simulink model "Microgrid_W"  (R2020a)
settings: Solver=ode15s  StartTime=0  StopTime=1440*1  MaxStep=1  RelTol=1e-3
libraries: simulink x4214, powerlib x685, simulink_extras x28, Microgrid_Library x18, powerlib_meascontrol x12
(part 37 of 48)

== system Microgrid_W/House 5 W1/Kettle/D4 ==
  Add : Sum  Inputs=+++
  Clock : Clock
  Compare To Zero : simulink/Logic and Bit Operations/Compare To Zero  relop=>  OutDataTypeStr=boolean
  Compare To Zero1 : simulink/Logic and Bit Operations/Compare To Zero  relop=>  OutDataTypeStr=boolean
  Compare To Zero2 : simulink/Logic and Bit Operations/Compare To Zero  relop=>  OutDataTypeStr=boolean
  Constant : Constant
  Constant{1..2,5,8} (4 alike) : Constant  Value=0
  Constant3 : Constant  Value=Jug_On_1
  Constant4 : Constant
  Constant6 : Constant  Value=Jug_On_2
  Constant7 : Constant
  Constant9 : Constant  Value=Jug_On_3
  Gain : Gain  Gain=t
  Interval Test : simulink/Logic and Bit Operations/Interval Test  IntervalClosedRight=on  uplimit=Jug_On_1+180+86400*3  IntervalClosedLeft=on  lowlimit=Jug_On_1+86400*3  OutDataTypeStr=boolean
  Interval Test1 : simulink/Logic and Bit Operations/Interval Test  IntervalClosedRight=on  uplimit=Jug_On_2+180+86400*3  IntervalClosedLeft=on  lowlimit=Jug_On_2+86400*3  OutDataTypeStr=boolean
  Interval Test2 : simulink/Logic and Bit Operations/Interval Test  IntervalClosedRight=on  uplimit=Jug_On_3+180+86400*3  IntervalClosedLeft=on  lowlimit=Jug_On_3+86400*3  OutDataTypeStr=boolean
  Switch{,1..5} (6 alike) : Switch  Criteria=u2 > Threshold  Threshold=0.5
  Out1 : Outport  VectorParamsAs1DForOutWhenUnconnected=off
  wires:
  Clock/1 -> Gain/1
  Interval Test/1 -> Switch/2
  Constant1/1 -> Switch3/3, Switch2/3, Switch/3
  Gain/1 -> Interval Test2/1, Interval Test1/1, Interval Test/1
  Constant3/1 -> Compare To Zero/1
  Constant/1 -> Switch1/1
  Constant2/1 -> Switch1/3
  Compare To Zero/1 -> Switch1/2
  Switch1/1 -> Switch/1
  Interval Test1/1 -> Switch2/2
  Interval Test2/1 -> Switch3/2
  Constant6/1 -> Compare To Zero1/1
  Constant4/1 -> Switch4/1
  Constant5/1 -> Switch4/3
  Compare To Zero1/1 -> Switch4/2
  Constant9/1 -> Compare To Zero2/1
  Constant7/1 -> Switch5/1
  Constant8/1 -> Switch5/3
  Compare To Zero2/1 -> Switch5/2
  Switch4/1 -> Switch2/1
  Switch5/1 -> Switch3/1
  Switch/1 -> Add/1
  Switch2/1 -> Add/2
  Switch3/1 -> Add/3
  Add/1 -> Out1/1

== system Microgrid_W/House 5 W1/Kettle/D5 ==
  Add : Sum  Inputs=+++
  Clock : Clock
  Compare To Zero : simulink/Logic and Bit Operations/Compare To Zero  relop=>  OutDataTypeStr=boolean
  Compare To Zero1 : simulink/Logic and Bit Operations/Compare To Zero  relop=>  OutDataTypeStr=boolean
  Compare To Zero2 : simulink/Logic and Bit Operations/Compare To Zero  relop=>  OutDataTypeStr=boolean
  Constant : Constant
  Constant{1..2,5,8} (4 alike) : Constant  Value=0
  Constant3 : Constant  Value=Jug_On_1
  Constant4 : Constant
  Constant6 : Constant  Value=Jug_On_2
  Constant7 : Constant
  Constant9 : Constant  Value=Jug_On_3
  Gain : Gain  Gain=t
  Interval Test : simulink/Logic and Bit Operations/Interval Test  IntervalClosedRight=on  uplimit=Jug_On_1+180+86400*4  IntervalClosedLeft=on  lowlimit=Jug_On_1+86400*4  OutDataTypeStr=boolean
  Interval Test1 : simulink/Logic and Bit Operations/Interval Test  IntervalClosedRight=on  uplimit=Jug_On_2+180+86400*4  IntervalClosedLeft=on  lowlimit=Jug_On_2+86400*4  OutDataTypeStr=boolean
  Interval Test2 : simulink/Logic and Bit Operations/Interval Test  IntervalClosedRight=on  uplimit=Jug_On_3+180+86400*4  IntervalClosedLeft=on  lowlimit=Jug_On_3+86400*4  OutDataTypeStr=boolean
  Switch{,1..5} (6 alike) : Switch  Criteria=u2 > Threshold  Threshold=0.5
  Out1 : Outport  VectorParamsAs1DForOutWhenUnconnected=off
  wires:
  Clock/1 -> Gain/1
  Add/1 -> Out1/1
  Switch3/1 -> Add/3
  Switch2/1 -> Add/2
  Switch/1 -> Add/1
  Switch5/1 -> Switch3/1
  Switch4/1 -> Switch2/1
  Compare To Zero2/1 -> Switch5/2
  Constant8/1 -> Switch5/3
  Constant7/1 -> Switch5/1
  Constant9/1 -> Compare To Zero2/1
  Compare To Zero1/1 -> Switch4/2
  Constant5/1 -> Switch4/3
  Constant4/1 -> Switch4/1
  Constant6/1 -> Compare To Zero1/1
  Interval Test2/1 -> Switch3/2
  Interval Test1/1 -> Switch2/2
  Switch1/1 -> Switch/1
  Compare To Zero/1 -> Switch1/2
  Constant2/1 -> Switch1/3
  Constant/1 -> Switch1/1
  Constant3/1 -> Compare To Zero/1
  Gain/1 -> Interval Test/1, Interval Test1/1, Interval Test2/1
  Constant1/1 -> Switch/3, Switch2/3, Switch3/3
  Interval Test/1 -> Switch/2

== system Microgrid_W/House 5 W1/Kettle/D6 ==
  Add : Sum  Inputs=+++
  Clock : Clock
  Compare To Zero : simulink/Logic and Bit Operations/Compare To Zero  relop=>  OutDataTypeStr=boolean
  Compare To Zero1 : simulink/Logic and Bit Operations/Compare To Zero  relop=>  OutDataTypeStr=boolean
  Compare To Zero2 : simulink/Logic and Bit Operations/Compare To Zero  relop=>  OutDataTypeStr=boolean
  Constant : Constant
  Constant{1..2,5,8} (4 alike) : Constant  Value=0
  Constant3 : Constant  Value=Jug_On_1
  Constant4 : Constant
  Constant6 : Constant  Value=Jug_On_2
  Constant7 : Constant
  Constant9 : Constant  Value=Jug_On_3
  Gain : Gain  Gain=t
  Interval Test : simulink/Logic and Bit Operations/Interval Test  IntervalClosedRight=on  uplimit=Jug_On_1+180+86400*5  IntervalClosedLeft=on  lowlimit=Jug_On_1+86400*5  OutDataTypeStr=boolean
  Interval Test1 : simulink/Logic and Bit Operations/Interval Test  IntervalClosedRight=on  uplimit=Jug_On_2+180+86400*5  IntervalClosedLeft=on  lowlimit=Jug_On_2+86400*5  OutDataTypeStr=boolean
  Interval Test2 : simulink/Logic and Bit Operations/Interval Test  IntervalClosedRight=on  uplimit=Jug_On_3+180+86400*5  IntervalClosedLeft=on  lowlimit=Jug_On_3+86400*5  OutDataTypeStr=boolean
  Switch{,1..5} (6 alike) : Switch  Criteria=u2 > Threshold  Threshold=0.5
  Out1 : Outport  VectorParamsAs1DForOutWhenUnconnected=off
  wires:
  Clock/1 -> Gain/1
  Interval Test/1 -> Switch/2
  Constant1/1 -> Switch3/3, Switch2/3, Switch/3
  Gain/1 -> Interval Test2/1, Interval Test1/1, Interval Test/1
  Constant3/1 -> Compare To Zero/1
  Constant/1 -> Switch1/1
  Constant2/1 -> Switch1/3
  Compare To Zero/1 -> Switch1/2
  Switch1/1 -> Switch/1
  Interval Test1/1 -> Switch2/2
  Interval Test2/1 -> Switch3/2
  Constant6/1 -> Compare To Zero1/1
  Constant4/1 -> Switch4/1
  Constant5/1 -> Switch4/3
  Compare To Zero1/1 -> Switch4/2
  Constant9/1 -> Compare To Zero2/1
  Constant7/1 -> Switch5/1
  Constant8/1 -> Switch5/3
  Compare To Zero2/1 -> Switch5/2
  Switch4/1 -> Switch2/1
  Switch5/1 -> Switch3/1
  Switch/1 -> Add/1
  Switch2/1 -> Add/2
  Switch3/1 -> Add/3
  Add/1 -> Out1/1

== system Microgrid_W/House 5 W1/Kettle/D7 ==
  Add : Sum  Inputs=+++
  Clock : Clock
  Compare To Zero : simulink/Logic and Bit Operations/Compare To Zero  relop=>  OutDataTypeStr=boolean
  Compare To Zero1 : simulink/Logic and Bit Operations/Compare To Zero  relop=>  OutDataTypeStr=boolean
  Compare To Zero2 : simulink/Logic and Bit Operations/Compare To Zero  relop=>  OutDataTypeStr=boolean
  Constant : Constant
  Constant{1..2,5,8} (4 alike) : Constant  Value=0
  Constant3 : Constant  Value=Jug_On_1
  Constant4 : Constant
  Constant6 : Constant  Value=Jug_On_2
  Constant7 : Constant
  Constant9 : Constant  Value=Jug_On_3
  Gain : Gain  Gain=t
  Interval Test : simulink/Logic and Bit Operations/Interval Test  IntervalClosedRight=on  uplimit=Jug_On_1+180+86400*6  IntervalClosedLeft=on  lowlimit=Jug_On_1+86400*6  OutDataTypeStr=boolean
  Interval Test1 : simulink/Logic and Bit Operations/Interval Test  IntervalClosedRight=on  uplimit=Jug_On_2+180+86400*6  IntervalClosedLeft=on  lowlimit=Jug_On_2+86400*6  OutDataTypeStr=boolean
  Interval Test2 : simulink/Logic and Bit Operations/Interval Test  IntervalClosedRight=on  uplimit=Jug_On_3+180+86400*6  IntervalClosedLeft=on  lowlimit=Jug_On_3+86400*6  OutDataTypeStr=boolean
  Switch{,1..5} (6 alike) : Switch  Criteria=u2 > Threshold  Threshold=0.5
  Out1 : Outport  VectorParamsAs1DForOutWhenUnconnected=off
  wires:
  Clock/1 -> Gain/1
  Add/1 -> Out1/1
  Switch3/1 -> Add/3
  Switch2/1 -> Add/2
  Switch/1 -> Add/1
  Switch5/1 -> Switch3/1
  Switch4/1 -> Switch2/1
  Compare To Zero2/1 -> Switch5/2
  Constant8/1 -> Switch5/3
  Constant7/1 -> Switch5/1
  Constant9/1 -> Compare To Zero2/1
  Compare To Zero1/1 -> Switch4/2
  Constant5/1 -> Switch4/3
  Constant4/1 -> Switch4/1
  Constant6/1 -> Compare To Zero1/1
  Interval Test2/1 -> Switch3/2
  Interval Test1/1 -> Switch2/2
  Switch1/1 -> Switch/1
  Compare To Zero/1 -> Switch1/2
  Constant2/1 -> Switch1/3
  Constant/1 -> Switch1/1
  Constant3/1 -> Compare To Zero/1
  Gain/1 -> Interval Test/1, Interval Test1/1, Interval Test2/1
  Constant1/1 -> Switch/3, Switch2/3, Switch3/3
  Interval Test/1 -> Switch/2

== system Microgrid_W/House 5 W1/Lamp 1/D1 ==
  Add : Sum
  Clock : Clock
  Constant : Constant
  Constant1 : Constant  Value=0
  Gain : Gain  Gain=t
  Interval Test : simulink/Logic and Bit Operations/Interval Test  IntervalClosedRight=on  uplimit=L1_Off_1  IntervalClosedLeft=on  lowlimit=L1_On_1  OutDataTypeStr=boolean
  Interval Test1 : simulink/Logic and Bit Operations/Interval Test  IntervalClosedRight=on  uplimit=L1_Off_2  IntervalClosedLeft=on  lowlimit=L1_On_2  OutDataTypeStr=boolean
  Switch : Switch  Criteria=u2 > Threshold  Threshold=0.5
  Switch1 : Switch  Criteria=u2 > Threshold  Threshold=0.5
  Out1 : Outport  VectorParamsAs1DForOutWhenUnconnected=off
  wires:
  Clock/1 -> Gain/1
  Interval Test/1 -> Switch/2
  Switch/1 -> Add/1
  Interval Test1/1 -> Switch1/2
  Add/1 -> Out1/1
  Constant1/1 -> Switch/3, Switch1/3
  Constant/1 -> Switch/1, Switch1/1
  Switch1/1 -> Add/2
  Gain/1 -> Interval Test1/1, Interval Test/1

== system Microgrid_W/House 5 W1/Lamp 1/D2 ==
  Add : Sum
  Clock : Clock
  Constant : Constant
  Constant1 : Constant  Value=0
  Gain : Gain  Gain=t
  Interval Test : simulink/Logic and Bit Operations/Interval Test  IntervalClosedRight=on  uplimit=L1_Off_1+86400  IntervalClosedLeft=on  lowlimit=L1_On_1+86400  OutDataTypeStr=boolean
  Interval Test1 : simulink/Logic and Bit Operations/Interval Test  IntervalClosedRight=on  uplimit=L1_Off_2+86400  IntervalClosedLeft=on  lowlimit=L1_On_2+86400  OutDataTypeStr=boolean
  Switch : Switch  Criteria=u2 > Threshold  Threshold=0.5
  Switch1 : Switch  Criteria=u2 > Threshold  Threshold=0.5
  Out1 : Outport  VectorParamsAs1DForOutWhenUnconnected=off
  wires:
  Clock/1 -> Gain/1
  Gain/1 -> Interval Test/1, Interval Test1/1
  Switch1/1 -> Add/2
  Constant/1 -> Switch1/1, Switch/1
  Constant1/1 -> Switch1/3, Switch/3
  Add/1 -> Out1/1
  Interval Test1/1 -> Switch1/2
  Switch/1 -> Add/1
  Interval Test/1 -> Switch/2

== system Microgrid_W/House 5 W1/Lamp 1/D3 ==
  Add : Sum
  Clock : Clock
  Constant : Constant
  Constant1 : Constant  Value=0
  Gain : Gain  Gain=t
  Interval Test : simulink/Logic and Bit Operations/Interval Test  IntervalClosedRight=on  uplimit=L1_Off_1+86400*2  IntervalClosedLeft=on  lowlimit=L1_On_1+86400*2  OutDataTypeStr=boolean
  Interval Test1 : simulink/Logic and Bit Operations/Interval Test  IntervalClosedRight=on  uplimit=L1_Off_2+86400*2  IntervalClosedLeft=on  lowlimit=L1_On_2+86400*2  OutDataTypeStr=boolean
  Switch : Switch  Criteria=u2 > Threshold  Threshold=0.5
  Switch1 : Switch  Criteria=u2 > Threshold  Threshold=0.5
  Out1 : Outport  VectorParamsAs1DForOutWhenUnconnected=off
  wires:
  Clock/1 -> Gain/1
  Interval Test/1 -> Switch/2
  Switch/1 -> Add/1
  Interval Test1/1 -> Switch1/2
  Add/1 -> Out1/1
  Constant1/1 -> Switch/3, Switch1/3
  Constant/1 -> Switch/1, Switch1/1
  Switch1/1 -> Add/2
  Gain/1 -> Interval Test1/1, Interval Test/1

== system Microgrid_W/House 5 W1/Lamp 1/D4 ==
  Add : Sum
  Clock : Clock
  Constant : Constant
  Constant1 : Constant  Value=0
  Gain : Gain  Gain=t
  Interval Test : simulink/Logic and Bit Operations/Interval Test  IntervalClosedRight=on  uplimit=L1_Off_1+86400*3  IntervalClosedLeft=on  lowlimit=L1_On_1+86400*3  OutDataTypeStr=boolean
  Interval Test1 : simulink/Logic and Bit Operations/Interval Test  IntervalClosedRight=on  uplimit=L1_Off_2+86400*3  IntervalClosedLeft=on  lowlimit=L1_On_2+86400*3  OutDataTypeStr=boolean
  Switch : Switch  Criteria=u2 > Threshold  Threshold=0.5
  Switch1 : Switch  Criteria=u2 > Threshold  Threshold=0.5
  Out1 : Outport  VectorParamsAs1DForOutWhenUnconnected=off
  wires:
  Clock/1 -> Gain/1
  ? -> Interval Test/1, Interval Test1/1
  Switch1/1 -> Add/2
  Constant/1 -> Switch1/1, Switch/1
  Constant1/1 -> Switch1/3, Switch/3
  Add/1 -> Out1/1
  Interval Test1/1 -> Switch1/2
  Switch/1 -> Add/1
  Interval Test/1 -> Switch/2

== system Microgrid_W/House 5 W1/Lamp 1/D5 ==
  Add : Sum
  Clock : Clock
  Constant : Constant
  Constant1 : Constant  Value=0
  Gain : Gain  Gain=t
  Interval Test : simulink/Logic and Bit Operations/Interval Test  IntervalClosedRight=on  uplimit=L1_Off_1+86400*4  IntervalClosedLeft=on  lowlimit=L1_On_1+86400*4  OutDataTypeStr=boolean
  Interval Test1 : simulink/Logic and Bit Operations/Interval Test  IntervalClosedRight=on  uplimit=L1_Off_2+86400*4  IntervalClosedLeft=on  lowlimit=L1_On_2+86400*4  OutDataTypeStr=boolean
  Switch : Switch  Criteria=u2 > Threshold  Threshold=0.5
  Switch1 : Switch  Criteria=u2 > Threshold  Threshold=0.5
  Out1 : Outport  VectorParamsAs1DForOutWhenUnconnected=off
  wires:
  Clock/1 -> Gain/1
  Interval Test/1 -> Switch/2
  Switch/1 -> Add/1
  Interval Test1/1 -> Switch1/2
  Add/1 -> Out1/1
  Constant1/1 -> Switch/3, Switch1/3
  Constant/1 -> Switch/1, Switch1/1
  Switch1/1 -> Add/2
  Gain/1 -> Interval Test1/1, Interval Test/1

== system Microgrid_W/House 5 W1/Lamp 1/D6 ==
  Add : Sum
  Clock : Clock
  Constant : Constant
  Constant1 : Constant  Value=0
  Gain : Gain  Gain=t
  Interval Test : simulink/Logic and Bit Operations/Interval Test  IntervalClosedRight=on  uplimit=L1_Off_1+86400*5  IntervalClosedLeft=on  lowlimit=L1_On_1+86400*5  OutDataTypeStr=boolean
  Interval Test1 : simulink/Logic and Bit Operations/Interval Test  IntervalClosedRight=on  uplimit=L1_Off_2+86400*5  IntervalClosedLeft=on  lowlimit=L1_On_2+86400*5  OutDataTypeStr=boolean
  Switch : Switch  Criteria=u2 > Threshold  Threshold=0.5
  Switch1 : Switch  Criteria=u2 > Threshold  Threshold=0.5
  Out1 : Outport  VectorParamsAs1DForOutWhenUnconnected=off
  wires:
  Clock/1 -> Gain/1
  Gain/1 -> Interval Test/1, Interval Test1/1
  Switch1/1 -> Add/2
  Constant/1 -> Switch1/1, Switch/1
  Constant1/1 -> Switch1/3, Switch/3
  Add/1 -> Out1/1
  Interval Test1/1 -> Switch1/2
  Switch/1 -> Add/1
  Interval Test/1 -> Switch/2

== system Microgrid_W/House 5 W1/Lamp 1/D7 ==
  Add : Sum
  Clock : Clock
  Constant : Constant
  Constant1 : Constant  Value=0
  Gain : Gain  Gain=t
  Interval Test : simulink/Logic and Bit Operations/Interval Test  IntervalClosedRight=on  uplimit=L1_Off_1+86400*6  IntervalClosedLeft=on  lowlimit=L1_On_1+86400*6  OutDataTypeStr=boolean
  Interval Test1 : simulink/Logic and Bit Operations/Interval Test  IntervalClosedRight=on  uplimit=L1_Off_2+86400*6  IntervalClosedLeft=on  lowlimit=L1_On_2+86400*6  OutDataTypeStr=boolean
  Switch : Switch  Criteria=u2 > Threshold  Threshold=0.5
  Switch1 : Switch  Criteria=u2 > Threshold  Threshold=0.5
  Out1 : Outport  VectorParamsAs1DForOutWhenUnconnected=off
  wires:
  Clock/1 -> Gain/1
  Interval Test/1 -> Switch/2
  Switch/1 -> Add/1
  Interval Test1/1 -> Switch1/2
  Add/1 -> Out1/1
  Constant1/1 -> Switch/3, Switch1/3
  Constant/1 -> Switch/1, Switch1/1
  Switch1/1 -> Add/2
  Gain/1 -> Interval Test1/1, Interval Test/1

== system Microgrid_W/House 5 W1/Lamp 2/D1 ==
  Add : Sum
  Clock : Clock
  Constant : Constant
  Constant1 : Constant  Value=0
  Gain : Gain  Gain=t
  Interval Test : simulink/Logic and Bit Operations/Interval Test  IntervalClosedRight=on  uplimit=L2_Off_1  IntervalClosedLeft=on  lowlimit=L2_On_1  OutDataTypeStr=boolean
  Interval Test1 : simulink/Logic and Bit Operations/Interval Test  IntervalClosedRight=on  uplimit=L2_Off_2  IntervalClosedLeft=on  lowlimit=L2_On_2  OutDataTypeStr=boolean
  Switch : Switch  Criteria=u2 > Threshold  Threshold=0.5
  Switch1 : Switch  Criteria=u2 > Threshold  Threshold=0.5
  Out1 : Outport  VectorParamsAs1DForOutWhenUnconnected=off
  wires:
  Clock/1 -> Gain/1
  Gain/1 -> Interval Test/1, Interval Test1/1
  Switch1/1 -> Add/2
  Constant/1 -> Switch1/1, Switch/1
  Constant1/1 -> Switch1/3, Switch/3
  Add/1 -> Out1/1
  Interval Test1/1 -> Switch1/2
  Switch/1 -> Add/1
  Interval Test/1 -> Switch/2

== system Microgrid_W/House 5 W1/Lamp 2/D2 ==
  Add : Sum
  Clock : Clock
  Constant : Constant
  Constant1 : Constant  Value=0
  Gain : Gain  Gain=t
  Interval Test : simulink/Logic and Bit Operations/Interval Test  IntervalClosedRight=on  uplimit=L2_Off_1+86400  IntervalClosedLeft=on  lowlimit=L2_On_1+86400  OutDataTypeStr=boolean
  Interval Test1 : simulink/Logic and Bit Operations/Interval Test  IntervalClosedRight=on  uplimit=L2_Off_2+86400  IntervalClosedLeft=on  lowlimit=L2_On_2+86400  OutDataTypeStr=boolean
  Switch : Switch  Criteria=u2 > Threshold  Threshold=0.5
  Switch1 : Switch  Criteria=u2 > Threshold  Threshold=0.5
  Out1 : Outport  VectorParamsAs1DForOutWhenUnconnected=off
  wires:
  Clock/1 -> Gain/1
  Interval Test/1 -> Switch/2
  Switch/1 -> Add/1
  Interval Test1/1 -> Switch1/2
  Add/1 -> Out1/1
  Constant1/1 -> Switch/3, Switch1/3
  Constant/1 -> Switch/1, Switch1/1
  Switch1/1 -> Add/2
  Gain/1 -> Interval Test1/1, Interval Test/1

== system Microgrid_W/House 5 W1/Lamp 2/D3 ==
  Add : Sum
  Clock : Clock
  Constant : Constant
  Constant1 : Constant  Value=0
  Gain : Gain  Gain=t
  Interval Test : simulink/Logic and Bit Operations/Interval Test  IntervalClosedRight=on  uplimit=L2_Off_1+86400*2  IntervalClosedLeft=on  lowlimit=L2_On_1+86400*2  OutDataTypeStr=boolean
  Interval Test1 : simulink/Logic and Bit Operations/Interval Test  IntervalClosedRight=on  uplimit=L2_Off_2+86400*2  IntervalClosedLeft=on  lowlimit=L2_On_2+86400*2  OutDataTypeStr=boolean
  Switch : Switch  Criteria=u2 > Threshold  Threshold=0.5
  Switch1 : Switch  Criteria=u2 > Threshold  Threshold=0.5
  Out1 : Outport  VectorParamsAs1DForOutWhenUnconnected=off
  wires:
  Clock/1 -> Gain/1
  Gain/1 -> Interval Test/1, Interval Test1/1
  Switch1/1 -> Add/2
  Constant/1 -> Switch1/1, Switch/1
  Constant1/1 -> Switch1/3, Switch/3
  Add/1 -> Out1/1
  Interval Test1/1 -> Switch1/2
  Switch/1 -> Add/1
  Interval Test/1 -> Switch/2

== system Microgrid_W/House 5 W1/Lamp 2/D4 ==
  Add : Sum
  Clock : Clock
  Constant : Constant
  Constant1 : Constant  Value=0
  Gain : Gain  Gain=t
  Interval Test : simulink/Logic and Bit Operations/Interval Test  IntervalClosedRight=on  uplimit=L2_Off_1+86400*3  IntervalClosedLeft=on  lowlimit=L2_On_1+86400*3  OutDataTypeStr=boolean
  Interval Test1 : simulink/Logic and Bit Operations/Interval Test  IntervalClosedRight=on  uplimit=L2_Off_2+86400*3  IntervalClosedLeft=on  lowlimit=L2_On_2+86400*3  OutDataTypeStr=boolean
  Switch : Switch  Criteria=u2 > Threshold  Threshold=0.5
  Switch1 : Switch  Criteria=u2 > Threshold  Threshold=0.5
  Out1 : Outport  VectorParamsAs1DForOutWhenUnconnected=off
  wires:
  Clock/1 -> Gain/1
  Interval Test/1 -> Switch/2
  Switch/1 -> Add/1
  Interval Test1/1 -> Switch1/2
  Add/1 -> Out1/1
  Constant1/1 -> Switch/3, Switch1/3
  Constant/1 -> Switch/1, Switch1/1
  Switch1/1 -> Add/2
  Gain/1 -> Interval Test1/1, Interval Test/1

== system Microgrid_W/House 5 W1/Lamp 2/D5 ==
  Add : Sum
  Clock : Clock
  Constant : Constant
  Constant1 : Constant  Value=0
  Gain : Gain  Gain=t
  Interval Test : simulink/Logic and Bit Operations/Interval Test  IntervalClosedRight=on  uplimit=L2_Off_1+86400*4  IntervalClosedLeft=on  lowlimit=L2_On_1+86400*4  OutDataTypeStr=boolean
  Interval Test1 : simulink/Logic and Bit Operations/Interval Test  IntervalClosedRight=on  uplimit=L2_Off_2+86400*4  IntervalClosedLeft=on  lowlimit=L2_On_2+86400*4  OutDataTypeStr=boolean
  Switch : Switch  Criteria=u2 > Threshold  Threshold=0.5
  Switch1 : Switch  Criteria=u2 > Threshold  Threshold=0.5
  Out1 : Outport  VectorParamsAs1DForOutWhenUnconnected=off
  wires:
  Clock/1 -> Gain/1
  Gain/1 -> Interval Test/1, Interval Test1/1
  Switch1/1 -> Add/2
  Constant/1 -> Switch1/1, Switch/1
  Constant1/1 -> Switch1/3, Switch/3
  Add/1 -> Out1/1
  Interval Test1/1 -> Switch1/2
  Switch/1 -> Add/1
  Interval Test/1 -> Switch/2

== system Microgrid_W/House 5 W1/Lamp 2/D6 ==
  Add : Sum
  Clock : Clock
  Constant : Constant
  Constant1 : Constant  Value=0
  Gain : Gain  Gain=t
  Interval Test : simulink/Logic and Bit Operations/Interval Test  IntervalClosedRight=on  uplimit=L2_Off_1+86400*5  IntervalClosedLeft=on  lowlimit=L2_On_1+86400*5  OutDataTypeStr=boolean
  Interval Test1 : simulink/Logic and Bit Operations/Interval Test  IntervalClosedRight=on  uplimit=L2_Off_2+86400*5  IntervalClosedLeft=on  lowlimit=L2_On_2+86400*5  OutDataTypeStr=boolean
  Switch : Switch  Criteria=u2 > Threshold  Threshold=0.5
  Switch1 : Switch  Criteria=u2 > Threshold  Threshold=0.5
  Out1 : Outport  VectorParamsAs1DForOutWhenUnconnected=off
  wires:
  Clock/1 -> Gain/1
  Interval Test/1 -> Switch/2
  Switch/1 -> Add/1
  Interval Test1/1 -> Switch1/2
  Add/1 -> Out1/1
  Constant1/1 -> Switch/3, Switch1/3
  Constant/1 -> Switch/1, Switch1/1
  Switch1/1 -> Add/2
  Gain/1 -> Interval Test1/1, Interval Test/1

== system Microgrid_W/House 5 W1/Lamp 2/D7 ==
  Add : Sum
  Clock : Clock
  Constant : Constant
  Constant1 : Constant  Value=0
  Gain : Gain  Gain=t
  Interval Test : simulink/Logic and Bit Operations/Interval Test  IntervalClosedRight=on  uplimit=L2_Off_1+86400*6  IntervalClosedLeft=on  lowlimit=L2_On_1+86400*6  OutDataTypeStr=boolean
  Interval Test1 : simulink/Logic and Bit Operations/Interval Test  IntervalClosedRight=on  uplimit=L2_Off_2+86400*6  IntervalClosedLeft=on  lowlimit=L2_On_2+86400*6  OutDataTypeStr=boolean
  Switch : Switch  Criteria=u2 > Threshold  Threshold=0.5
  Switch1 : Switch  Criteria=u2 > Threshold  Threshold=0.5
  Out1 : Outport  VectorParamsAs1DForOutWhenUnconnected=off
  wires:
  Clock/1 -> Gain/1
  Gain/1 -> Interval Test/1, Interval Test1/1
  Switch1/1 -> Add/2
  Constant/1 -> Switch1/1, Switch/1
  Constant1/1 -> Switch1/3, Switch/3
  Add/1 -> Out1/1
  Interval Test1/1 -> Switch1/2
  Switch/1 -> Add/1
  Interval Test/1 -> Switch/2

== system Microgrid_W/House 5 W1/Lamp 3/D1 ==
  Add : Sum
  Clock : Clock
  Constant : Constant
  Constant1 : Constant  Value=0
  Gain : Gain  Gain=t
  Interval Test : simulink/Logic and Bit Operations/Interval Test  IntervalClosedRight=on  uplimit=L3_Off_1  IntervalClosedLeft=on  lowlimit=L3_On_1  OutDataTypeStr=boolean
  Interval Test1 : simulink/Logic and Bit Operations/Interval Test  IntervalClosedRight=on  uplimit=L3_Off_2  IntervalClosedLeft=on  lowlimit=L3_On_2  OutDataTypeStr=boolean
  Switch : Switch  Criteria=u2 > Threshold  Threshold=0.5
  Switch1 : Switch  Criteria=u2 > Threshold  Threshold=0.5
  Out1 : Outport  VectorParamsAs1DForOutWhenUnconnected=off
  wires:
  Clock/1 -> Gain/1
  Interval Test/1 -> Switch/2
  Switch/1 -> Add/1
  Interval Test1/1 -> Switch1/2
  Add/1 -> Out1/1
  Constant1/1 -> Switch/3, Switch1/3
  Constant/1 -> Switch/1, Switch1/1
  Switch1/1 -> Add/2
  Gain/1 -> Interval Test1/1, Interval Test/1

== system Microgrid_W/House 5 W1/Lamp 3/D2 ==
  Add : Sum
  Clock : Clock
  Constant : Constant
  Constant1 : Constant  Value=0
  Gain : Gain  Gain=t
  Interval Test : simulink/Logic and Bit Operations/Interval Test  IntervalClosedRight=on  uplimit=L3_Off_1+86400  IntervalClosedLeft=on  lowlimit=L3_On_1+86400  OutDataTypeStr=boolean
  Interval Test1 : simulink/Logic and Bit Operations/Interval Test  IntervalClosedRight=on  uplimit=L3_Off_2+86400  IntervalClosedLeft=on  lowlimit=L3_On_2+86400  OutDataTypeStr=boolean
  Switch : Switch  Criteria=u2 > Threshold  Threshold=0.5
  Switch1 : Switch  Criteria=u2 > Threshold  Threshold=0.5
  Out1 : Outport  VectorParamsAs1DForOutWhenUnconnected=off
  wires:
  Clock/1 -> Gain/1
  Gain/1 -> Interval Test/1, Interval Test1/1
  Switch1/1 -> Add/2
  Constant/1 -> Switch1/1, Switch/1
  Constant1/1 -> Switch1/3, Switch/3
  Add/1 -> Out1/1
  Interval Test1/1 -> Switch1/2
  Switch/1 -> Add/1
  Interval Test/1 -> Switch/2

== system Microgrid_W/House 5 W1/Lamp 3/D3 ==
  Add : Sum
  Clock : Clock
  Constant : Constant
  Constant1 : Constant  Value=0
  Gain : Gain  Gain=t
  Interval Test : simulink/Logic and Bit Operations/Interval Test  IntervalClosedRight=on  uplimit=L3_Off_1+86400*2  IntervalClosedLeft=on  lowlimit=L3_On_1+86400*2  OutDataTypeStr=boolean
  Interval Test1 : simulink/Logic and Bit Operations/Interval Test  IntervalClosedRight=on  uplimit=L3_Off_2+86400*2  IntervalClosedLeft=on  lowlimit=L3_On_2+86400*2  OutDataTypeStr=boolean
  Switch : Switch  Criteria=u2 > Threshold  Threshold=0.5
  Switch1 : Switch  Criteria=u2 > Threshold  Threshold=0.5
  Out1 : Outport  VectorParamsAs1DForOutWhenUnconnected=off
  wires:
  Clock/1 -> Gain/1
  Interval Test/1 -> Switch/2
  Switch/1 -> Add/1
  Interval Test1/1 -> Switch1/2
  Add/1 -> Out1/1
  Constant1/1 -> Switch/3, Switch1/3
  Constant/1 -> Switch/1, Switch1/1
  Switch1/1 -> Add/2
  Gain/1 -> Interval Test1/1, Interval Test/1

== system Microgrid_W/House 5 W1/Lamp 3/D4 ==
  Add : Sum
  Clock : Clock
  Constant : Constant
  Constant1 : Constant  Value=0
  Gain : Gain  Gain=t
  Interval Test : simulink/Logic and Bit Operations/Interval Test  IntervalClosedRight=on  uplimit=L3_Off_1+86400*3  IntervalClosedLeft=on  lowlimit=L3_On_1+86400*3  OutDataTypeStr=boolean
  Interval Test1 : simulink/Logic and Bit Operations/Interval Test  IntervalClosedRight=on  uplimit=L3_Off_2+86400*3  IntervalClosedLeft=on  lowlimit=L3_On_2+86400*3  OutDataTypeStr=boolean
  Switch : Switch  Criteria=u2 > Threshold  Threshold=0.5
  Switch1 : Switch  Criteria=u2 > Threshold  Threshold=0.5
  Out1 : Outport  VectorParamsAs1DForOutWhenUnconnected=off
  wires:
  Clock/1 -> Gain/1
  Gain/1 -> Interval Test/1, Interval Test1/1
  Switch1/1 -> Add/2
  Constant/1 -> Switch1/1, Switch/1
  Constant1/1 -> Switch1/3, Switch/3
  Add/1 -> Out1/1
  Interval Test1/1 -> Switch1/2
  Switch/1 -> Add/1
  Interval Test/1 -> Switch/2

== system Microgrid_W/House 5 W1/Lamp 3/D5 ==
  Add : Sum
  Clock : Clock
  Constant : Constant
  Constant1 : Constant  Value=0
  Gain : Gain  Gain=t
  Interval Test : simulink/Logic and Bit Operations/Interval Test  IntervalClosedRight=on  uplimit=L3_Off_1+86400*4  IntervalClosedLeft=on  lowlimit=L3_On_1+86400*4  OutDataTypeStr=boolean
  Interval Test1 : simulink/Logic and Bit Operations/Interval Test  IntervalClosedRight=on  uplimit=L3_Off_2+86400*4  IntervalClosedLeft=on  lowlimit=L3_On_2+86400*4  OutDataTypeStr=boolean
  Switch : Switch  Criteria=u2 > Threshold  Threshold=0.5
  Switch1 : Switch  Criteria=u2 > Threshold  Threshold=0.5
  Out1 : Outport  VectorParamsAs1DForOutWhenUnconnected=off
  wires:
  Clock/1 -> Gain/1
  Interval Test/1 -> Switch/2
  Switch/1 -> Add/1
  Interval Test1/1 -> Switch1/2
  Add/1 -> Out1/1
  Constant1/1 -> Switch/3, Switch1/3
  Constant/1 -> Switch/1, Switch1/1
  Switch1/1 -> Add/2
  Gain/1 -> Interval Test1/1, Interval Test/1

== system Microgrid_W/House 5 W1/Lamp 3/D6 ==
  Add : Sum
  Clock : Clock
  Constant : Constant
  Constant1 : Constant  Value=0
  Gain : Gain  Gain=t
  Interval Test : simulink/Logic and Bit Operations/Interval Test  IntervalClosedRight=on  uplimit=L3_Off_1+86400*5  IntervalClosedLeft=on  lowlimit=L3_On_1+86400*5  OutDataTypeStr=boolean
  Interval Test1 : simulink/Logic and Bit Operations/Interval Test  IntervalClosedRight=on  uplimit=L3_Off_2+86400*5  IntervalClosedLeft=on  lowlimit=L3_On_2+86400*5  OutDataTypeStr=boolean
  Switch : Switch  Criteria=u2 > Threshold  Threshold=0.5
  Switch1 : Switch  Criteria=u2 > Threshold  Threshold=0.5
  Out1 : Outport  VectorParamsAs1DForOutWhenUnconnected=off
  wires:
  Clock/1 -> Gain/1
  Gain/1 -> Interval Test/1, Interval Test1/1
  Switch1/1 -> Add/2
  Constant/1 -> Switch1/1, Switch/1
  Constant1/1 -> Switch1/3, Switch/3
  Add/1 -> Out1/1
  Interval Test1/1 -> Switch1/2
  Switch/1 -> Add/1
  Interval Test/1 -> Switch/2

== system Microgrid_W/House 5 W1/Lamp 3/D7 ==
  Add : Sum
  Clock : Clock
  Constant : Constant
  Constant1 : Constant  Value=0
  Gain : Gain  Gain=t
  Interval Test : simulink/Logic and Bit Operations/Interval Test  IntervalClosedRight=on  uplimit=L3_Off_1+86400*6  IntervalClosedLeft=on  lowlimit=L3_On_1+86400*6  OutDataTypeStr=boolean
  Interval Test1 : simulink/Logic and Bit Operations/Interval Test  IntervalClosedRight=on  uplimit=L3_Off_2+86400*6  IntervalClosedLeft=on  lowlimit=L3_On_2+86400*6  OutDataTypeStr=boolean
  Switch : Switch  Criteria=u2 > Threshold  Threshold=0.5
  Switch1 : Switch  Criteria=u2 > Threshold  Threshold=0.5
  Out1 : Outport  VectorParamsAs1DForOutWhenUnconnected=off
  wires:
  Clock/1 -> Gain/1
  Interval Test/1 -> Switch/2
  Switch/1 -> Add/1
  Interval Test1/1 -> Switch1/2
  Add/1 -> Out1/1
  Constant1/1 -> Switch/3, Switch1/3
  Constant/1 -> Switch/1, Switch1/1
  Switch1/1 -> Add/2
  Gain/1 -> Interval Test1/1, Interval Test/1

== system Microgrid_W/House 5 W1/Laptop_Charger/D1 ==
  Add : Sum
  Clock : Clock
  Constant : Constant
  Constant1 : Constant  Value=0
  Gain : Gain  Gain=t
  Interval Test : simulink/Logic and Bit Operations/Interval Test  IntervalClosedRight=on  uplimit=Laptop_C_2_Off_a  IntervalClosedLeft=on  lowlimit=Laptop_C_2_On_a  OutDataTypeStr=boolean
  Interval Test1 : simulink/Logic and Bit Operations/Interval Test  IntervalClosedRight=on  uplimit=Laptop_C_2_Off_b  IntervalClosedLeft=on  lowlimit=Laptop_C_2_On_b  OutDataTypeStr=boolean
  Switch : Switch  Criteria=u2 > Threshold  Threshold=0.5
  Switch1 : Switch  Criteria=u2 > Threshold  Threshold=0.5
  Out1 : Outport  VectorParamsAs1DForOutWhenUnconnected=off
  wires:
  Clock/1 -> Gain/1
  Interval Test/1 -> Switch/2
  Switch/1 -> Add/1
  Interval Test1/1 -> Switch1/2
  Add/1 -> Out1/1
  Constant1/1 -> Switch/3, Switch1/3
  Constant/1 -> Switch/1, Switch1/1
  Switch1/1 -> Add/2
  Gain/1 -> Interval Test1/1, Interval Test/1

== system Microgrid_W/House 5 W1/Laptop_Charger/D10 ==
  Clock : Clock
  Constant : Constant
  Constant1 : Constant  Value=0
  Gain : Gain  Gain=t
  Interval Test : simulink/Logic and Bit Operations/Interval Test  IntervalClosedRight=on  uplimit=Laptop_C_1_Off_a+86400*2  IntervalClosedLeft=on  lowlimit=Laptop_C_1_On_a+86400*2  OutDataTypeStr=boolean
  Switch : Switch  Criteria=u2 > Threshold  Threshold=0.5
  Out1 : Outport  VectorParamsAs1DForOutWhenUnconnected=off
  wires:
  Clock/1 -> Gain/1
  Gain/1 -> Interval Test/1
  Constant/1 -> Switch/1
  Constant1/1 -> Switch/3
  Switch/1 -> Out1/1
  Interval Test/1 -> Switch/2

== system Microgrid_W/House 5 W1/Laptop_Charger/D11 ==
  Clock : Clock
  Constant : Constant
  Constant1 : Constant  Value=0
  Gain : Gain  Gain=t
  Interval Test : simulink/Logic and Bit Operations/Interval Test  IntervalClosedRight=on  uplimit=Laptop_C_1_Off_a+86400*3  IntervalClosedLeft=on  lowlimit=Laptop_C_1_On_a+86400*3  OutDataTypeStr=boolean
  Switch : Switch  Criteria=u2 > Threshold  Threshold=0.5
  Out1 : Outport  VectorParamsAs1DForOutWhenUnconnected=off
  wires:
  Clock/1 -> Gain/1
  Interval Test/1 -> Switch/2
  Switch/1 -> Out1/1
  Constant1/1 -> Switch/3
  Constant/1 -> Switch/1
  Gain/1 -> Interval Test/1

== system Microgrid_W/House 5 W1/Laptop_Charger/D12 ==
  Clock : Clock
  Constant : Constant
  Constant1 : Constant  Value=0
  Gain : Gain  Gain=t
  Interval Test : simulink/Logic and Bit Operations/Interval Test  IntervalClosedRight=on  uplimit=Laptop_C_1_Off_a+86400*4  IntervalClosedLeft=on  lowlimit=Laptop_C_1_On_a+86400*4  OutDataTypeStr=boolean
  Switch : Switch  Criteria=u2 > Threshold  Threshold=0.5
  Out1 : Outport  VectorParamsAs1DForOutWhenUnconnected=off
  wires:
  Clock/1 -> Gain/1
  Gain/1 -> Interval Test/1
  Constant/1 -> Switch/1
  Constant1/1 -> Switch/3
  Switch/1 -> Out1/1
  Interval Test/1 -> Switch/2

== system Microgrid_W/House 5 W1/Laptop_Charger/D13 ==
  Clock : Clock
  Constant : Constant
  Constant1 : Constant  Value=0
  Gain : Gain  Gain=t
  Interval Test : simulink/Logic and Bit Operations/Interval Test  IntervalClosedRight=on  uplimit=Laptop_C_1_Off_a+86400*5  IntervalClosedLeft=on  lowlimit=Laptop_C_1_On_a+86400*5  OutDataTypeStr=boolean
  Switch : Switch  Criteria=u2 > Threshold  Threshold=0.5
  Out1 : Outport  VectorParamsAs1DForOutWhenUnconnected=off
  wires:
  Clock/1 -> Gain/1
  Interval Test/1 -> Switch/2
  Switch/1 -> Out1/1
  Constant1/1 -> Switch/3
  Constant/1 -> Switch/1
  Gain/1 -> Interval Test/1

== system Microgrid_W/House 5 W1/Laptop_Charger/D14 ==
  Clock : Clock
  Constant : Constant
  Constant1 : Constant  Value=0
  Gain : Gain  Gain=t
  Interval Test : simulink/Logic and Bit Operations/Interval Test  IntervalClosedRight=on  uplimit=Laptop_C_1_Off_a+86400*6  IntervalClosedLeft=on  lowlimit=Laptop_C_1_On_a+86400*6  OutDataTypeStr=boolean
  Switch : Switch  Criteria=u2 > Threshold  Threshold=0.5
  Out1 : Outport  VectorParamsAs1DForOutWhenUnconnected=off
  wires:
  Clock/1 -> Gain/1
  Gain/1 -> Interval Test/1
  Constant/1 -> Switch/1
  Constant1/1 -> Switch/3
  Switch/1 -> Out1/1
  Interval Test/1 -> Switch/2

== system Microgrid_W/House 5 W1/Laptop_Charger/D2 ==
  Add : Sum
  Clock : Clock
  Constant : Constant
  Constant1 : Constant  Value=0
  Gain : Gain  Gain=t
  Interval Test : simulink/Logic and Bit Operations/Interval Test  IntervalClosedRight=on  uplimit=Laptop_C_2_Off_a+86400  IntervalClosedLeft=on  lowlimit=Laptop_C_2_On_a+86400  OutDataTypeStr=boolean
  Interval Test1 : simulink/Logic and Bit Operations/Interval Test  IntervalClosedRight=on  uplimit=Laptop_C_2_Off_b+86400  IntervalClosedLeft=on  lowlimit=Laptop_C_2_On_b+86400  OutDataTypeStr=boolean
  Switch : Switch  Criteria=u2 > Threshold  Threshold=0.5
  Switch1 : Switch  Criteria=u2 > Threshold  Threshold=0.5
  Out1 : Outport  VectorParamsAs1DForOutWhenUnconnected=off
  wires:
  Clock/1 -> Gain/1
  Gain/1 -> Interval Test/1, Interval Test1/1
  Switch1/1 -> Add/2
  Constant/1 -> Switch1/1, Switch/1
  Constant1/1 -> Switch1/3, Switch/3
  Add/1 -> Out1/1
  Interval Test1/1 -> Switch1/2
  Switch/1 -> Add/1
  Interval Test/1 -> Switch/2

== system Microgrid_W/House 5 W1/Laptop_Charger/D3 ==
  Add : Sum
  Clock : Clock
  Constant : Constant
  Constant1 : Constant  Value=0
  Gain : Gain  Gain=t
  Interval Test : simulink/Logic and Bit Operations/Interval Test  IntervalClosedRight=on  uplimit=Laptop_C_2_Off_a+86400*2  IntervalClosedLeft=on  lowlimit=Laptop_C_2_On_a+86400*2  OutDataTypeStr=boolean
  Interval Test1 : simulink/Logic and Bit Operations/Interval Test  IntervalClosedRight=on  uplimit=Laptop_C_2_Off_b+86400*2  IntervalClosedLeft=on  lowlimit=Laptop_C_2_On_b+86400*2  OutDataTypeStr=boolean
  Switch : Switch  Criteria=u2 > Threshold  Threshold=0.5
  Switch1 : Switch  Criteria=u2 > Threshold  Threshold=0.5
  Out1 : Outport  VectorParamsAs1DForOutWhenUnconnected=off
  wires:
  Clock/1 -> Gain/1
  Interval Test/1 -> Switch/2
  Switch/1 -> Add/1
  Interval Test1/1 -> Switch1/2
  Add/1 -> Out1/1
  Constant1/1 -> Switch/3, Switch1/3
  Constant/1 -> Switch/1, Switch1/1
  Switch1/1 -> Add/2
  Gain/1 -> Interval Test1/1, Interval Test/1

== system Microgrid_W/House 5 W1/Laptop_Charger/D4 ==
  Add : Sum
  Clock : Clock
  Constant : Constant
  Constant1 : Constant  Value=0
  Gain : Gain  Gain=t
  Interval Test : simulink/Logic and Bit Operations/Interval Test  IntervalClosedRight=on  uplimit=Laptop_C_2_Off_a+86400*3  IntervalClosedLeft=on  lowlimit=Laptop_C_2_On_a+86400*3  OutDataTypeStr=boolean
  Interval Test1 : simulink/Logic and Bit Operations/Interval Test  IntervalClosedRight=on  uplimit=Laptop_C_2_Off_b+86400*3  IntervalClosedLeft=on  lowlimit=Laptop_C_2_On_b+86400*3  OutDataTypeStr=boolean
  Switch : Switch  Criteria=u2 > Threshold  Threshold=0.5
  Switch1 : Switch  Criteria=u2 > Threshold  Threshold=0.5
  Out1 : Outport  VectorParamsAs1DForOutWhenUnconnected=off
  wires:
  Clock/1 -> Gain/1
  Gain/1 -> Interval Test/1, Interval Test1/1
  Switch1/1 -> Add/2
  Constant/1 -> Switch1/1, Switch/1
  Constant1/1 -> Switch1/3, Switch/3
  Add/1 -> Out1/1
  Interval Test1/1 -> Switch1/2
  Switch/1 -> Add/1
  Interval Test/1 -> Switch/2

== system Microgrid_W/House 5 W1/Laptop_Charger/D5 ==
  Add : Sum
  Clock : Clock
  Constant : Constant
  Constant1 : Constant  Value=0
  Gain : Gain  Gain=t
  Interval Test : simulink/Logic and Bit Operations/Interval Test  IntervalClosedRight=on  uplimit=Laptop_C_2_Off_a+86400*4  IntervalClosedLeft=on  lowlimit=Laptop_C_2_On_a+86400*4  OutDataTypeStr=boolean
  Interval Test1 : simulink/Logic and Bit Operations/Interval Test  IntervalClosedRight=on  uplimit=Laptop_C_2_Off_b+86400*4  IntervalClosedLeft=on  lowlimit=Laptop_C_2_On_b+86400*4  OutDataTypeStr=boolean
  Switch : Switch  Criteria=u2 > Threshold  Threshold=0.5
  Switch1 : Switch  Criteria=u2 > Threshold  Threshold=0.5
  Out1 : Outport  VectorParamsAs1DForOutWhenUnconnected=off
  wires:
  Clock/1 -> Gain/1
  Interval Test/1 -> Switch/2
  Switch/1 -> Add/1
  Interval Test1/1 -> Switch1/2
  Add/1 -> Out1/1
  Constant1/1 -> Switch/3, Switch1/3
  Constant/1 -> Switch/1, Switch1/1
  Switch1/1 -> Add/2
  Gain/1 -> Interval Test1/1, Interval Test/1

== system Microgrid_W/House 5 W1/Laptop_Charger/D6 ==
  Add : Sum
  Clock : Clock
  Constant : Constant
  Constant1 : Constant  Value=0
  Gain : Gain  Gain=t
  Interval Test : simulink/Logic and Bit Operations/Interval Test  IntervalClosedRight=on  uplimit=Laptop_C_2_Off_a+86400*5  IntervalClosedLeft=on  lowlimit=Laptop_C_2_On_a+86400*5  OutDataTypeStr=boolean
  Interval Test1 : simulink/Logic and Bit Operations/Interval Test  IntervalClosedRight=on  uplimit=Laptop_C_2_Off_b+86400*5  IntervalClosedLeft=on  lowlimit=Laptop_C_2_On_b+86400*5  OutDataTypeStr=boolean
  Switch : Switch  Criteria=u2 > Threshold  Threshold=0.5
  Switch1 : Switch  Criteria=u2 > Threshold  Threshold=0.5
  Out1 : Outport  VectorParamsAs1DForOutWhenUnconnected=off
  wires:
  Clock/1 -> Gain/1
  Gain/1 -> Interval Test/1, Interval Test1/1
  Switch1/1 -> Add/2
  Constant/1 -> Switch1/1, Switch/1
  Constant1/1 -> Switch1/3, Switch/3
  Add/1 -> Out1/1
  Interval Test1/1 -> Switch1/2
  Switch/1 -> Add/1
  Interval Test/1 -> Switch/2

== system Microgrid_W/House 5 W1/Laptop_Charger/D7 ==
  Add : Sum
  Clock : Clock
  Constant : Constant
  Constant1 : Constant  Value=0
  Gain : Gain  Gain=t
  Interval Test : simulink/Logic and Bit Operations/Interval Test  IntervalClosedRight=on  uplimit=Laptop_C_2_Off_a+86400*6  IntervalClosedLeft=on  lowlimit=Laptop_C_2_On_a+86400*6  OutDataTypeStr=boolean
  Interval Test1 : simulink/Logic and Bit Operations/Interval Test  IntervalClosedRight=on  uplimit=Laptop_C_2_Off_b+86400*6  IntervalClosedLeft=on  lowlimit=Laptop_C_2_On_b+86400*6  OutDataTypeStr=boolean
  Switch : Switch  Criteria=u2 > Threshold  Threshold=0.5
  Switch1 : Switch  Criteria=u2 > Threshold  Threshold=0.5
  Out1 : Outport  VectorParamsAs1DForOutWhenUnconnected=off
  wires:
  Clock/1 -> Gain/1
  Interval Test/1 -> Switch/2
  Switch/1 -> Add/1
  Interval Test1/1 -> Switch1/2
  Add/1 -> Out1/1
  Constant1/1 -> Switch/3, Switch1/3
  Constant/1 -> Switch/1, Switch1/1
  Switch1/1 -> Add/2
  Gain/1 -> Interval Test1/1, Interval Test/1

== system Microgrid_W/House 5 W1/Laptop_Charger/D8 ==
  Clock : Clock
  Constant : Constant
  Constant1 : Constant  Value=0
  Gain : Gain  Gain=t
  Interval Test : simulink/Logic and Bit Operations/Interval Test  IntervalClosedRight=on  uplimit=Laptop_C_1_Off_a  IntervalClosedLeft=on  lowlimit=Laptop_C_1_On_a  OutDataTypeStr=boolean
  Switch : Switch  Criteria=u2 > Threshold  Threshold=0.5
  Out1 : Outport  VectorParamsAs1DForOutWhenUnconnected=off
  wires:
  Clock/1 -> Gain/1
  Gain/1 -> Interval Test/1
  Constant/1 -> Switch/1
  Constant1/1 -> Switch/3
  Switch/1 -> Out1/1
  Interval Test/1 -> Switch/2

== system Microgrid_W/House 5 W1/Laptop_Charger/D9 ==
  Clock : Clock
  Constant : Constant
  Constant1 : Constant  Value=0
  Gain : Gain  Gain=t
  Interval Test : simulink/Logic and Bit Operations/Interval Test  IntervalClosedRight=on  uplimit=Laptop_C_1_Off_a+86400  IntervalClosedLeft=on  lowlimit=Laptop_C_1_On_a+86400  OutDataTypeStr=boolean
  Switch : Switch  Criteria=u2 > Threshold  Threshold=0.5
  Out1 : Outport  VectorParamsAs1DForOutWhenUnconnected=off
  wires:
  Clock/1 -> Gain/1
  Interval Test/1 -> Switch/2
  Switch/1 -> Out1/1
  Constant1/1 -> Switch/3
  Constant/1 -> Switch/1
  Gain/1 -> Interval Test/1

== system Microgrid_W/House 5 W1/Light 1/D1 ==
  Add : Sum
  Clock : Clock
  Constant : Constant
  Constant1 : Constant  Value=0
  Gain : Gain  Gain=t
  Interval Test : simulink/Logic and Bit Operations/Interval Test  IntervalClosedRight=on  uplimit=K_L1_Off_1  IntervalClosedLeft=on  lowlimit=K_L1_On_1  OutDataTypeStr=boolean
  Interval Test1 : simulink/Logic and Bit Operations/Interval Test  IntervalClosedRight=on  uplimit=K_L1_Off_2  IntervalClosedLeft=on  lowlimit=K_L1_On_2  OutDataTypeStr=boolean
  Switch : Switch  Criteria=u2 > Threshold  Threshold=0.5
  Switch1 : Switch  Criteria=u2 > Threshold  Threshold=0.5
  Out1 : Outport  VectorParamsAs1DForOutWhenUnconnected=off
  wires:
  Gain/1 -> Interval Test1/1, Interval Test/1
  Interval Test/1 -> Switch/2
  Switch/1 -> Add/1
  Interval Test1/1 -> Switch1/2
  Add/1 -> Out1/1
  Constant1/1 -> Switch/3, Switch1/3
  Constant/1 -> Switch/1, Switch1/1
  Switch1/1 -> Add/2
  Clock/1 -> Gain/1

== system Microgrid_W/House 5 W1/Light 1/D2 ==
  Add : Sum
  Clock1 : Clock
  Constant : Constant
  Constant1 : Constant  Value=0
  Gain : Gain  Gain=t
  Interval Test : simulink/Logic and Bit Operations/Interval Test  IntervalClosedRight=on  uplimit=K_L1_Off_1+86400  IntervalClosedLeft=on  lowlimit=K_L1_On_1+86400  OutDataTypeStr=boolean
  Interval Test1 : simulink/Logic and Bit Operations/Interval Test  IntervalClosedRight=on  uplimit=K_L1_Off_2+86400  IntervalClosedLeft=on  lowlimit=K_L1_On_2+86400  OutDataTypeStr=boolean
  Switch : Switch  Criteria=u2 > Threshold  Threshold=0.5
  Switch1 : Switch  Criteria=u2 > Threshold  Threshold=0.5
  Out1 : Outport  VectorParamsAs1DForOutWhenUnconnected=off
  wires:
  Clock1/1 -> Gain/1
  Gain/1 -> Interval Test/1, Interval Test1/1
  Switch1/1 -> Add/2
  Constant/1 -> Switch1/1, Switch/1
  Constant1/1 -> Switch1/3, Switch/3
  Add/1 -> Out1/1
  Interval Test1/1 -> Switch1/2
  Switch/1 -> Add/1
  Interval Test/1 -> Switch/2

== system Microgrid_W/House 5 W1/Light 1/D3 ==
  Add : Sum
  Clock1 : Clock
  Constant : Constant
  Constant1 : Constant  Value=0
  Gain : Gain  Gain=t
  Interval Test : simulink/Logic and Bit Operations/Interval Test  IntervalClosedRight=on  uplimit=K_L1_Off_1+86400*2  IntervalClosedLeft=on  lowlimit=K_L1_On_1+86400*2  OutDataTypeStr=boolean
  Interval Test1 : simulink/Logic and Bit Operations/Interval Test  IntervalClosedRight=on  uplimit=K_L1_Off_2+86400*2  IntervalClosedLeft=on  lowlimit=K_L1_On_2+86400*2  OutDataTypeStr=boolean
  Switch : Switch  Criteria=u2 > Threshold  Threshold=0.5
  Switch1 : Switch  Criteria=u2 > Threshold  Threshold=0.5
  Out1 : Outport  VectorParamsAs1DForOutWhenUnconnected=off
  wires:
  Clock1/1 -> Gain/1
  Interval Test/1 -> Switch/2
  Switch/1 -> Add/1
  Interval Test1/1 -> Switch1/2
  Add/1 -> Out1/1
  Constant1/1 -> Switch/3, Switch1/3
  Constant/1 -> Switch/1, Switch1/1
  Switch1/1 -> Add/2
  Gain/1 -> Interval Test1/1, Interval Test/1

== system Microgrid_W/House 5 W1/Light 1/D4 ==
  Add : Sum
  Clock : Clock
  Constant : Constant
  Constant1 : Constant  Value=0
  Gain : Gain  Gain=t
  Interval Test : simulink/Logic and Bit Operations/Interval Test  IntervalClosedRight=on  uplimit=K_L1_Off_1+86400*3  IntervalClosedLeft=on  lowlimit=K_L1_On_1+86400*3  OutDataTypeStr=boolean
  Interval Test1 : simulink/Logic and Bit Operations/Interval Test  IntervalClosedRight=on  uplimit=K_L1_Off_2+86400*3  IntervalClosedLeft=on  lowlimit=K_L1_On_2+86400*3  OutDataTypeStr=boolean
  Switch : Switch  Criteria=u2 > Threshold  Threshold=0.5
  Switch1 : Switch  Criteria=u2 > Threshold  Threshold=0.5
  Out1 : Outport  VectorParamsAs1DForOutWhenUnconnected=off
  wires:
  Clock/1 -> Gain/1
  Gain/1 -> Interval Test/1, Interval Test1/1
  Switch1/1 -> Add/2
  Constant/1 -> Switch1/1, Switch/1
  Constant1/1 -> Switch1/3, Switch/3
  Add/1 -> Out1/1
  Interval Test1/1 -> Switch1/2
  Switch/1 -> Add/1
  Interval Test/1 -> Switch/2

== system Microgrid_W/House 5 W1/Light 1/D5 ==
  Add : Sum
  Clock : Clock
  Constant : Constant
  Constant1 : Constant  Value=0
  Gain : Gain  Gain=t
  Interval Test : simulink/Logic and Bit Operations/Interval Test  IntervalClosedRight=on  uplimit=K_L1_Off_1+86400*4  IntervalClosedLeft=on  lowlimit=K_L1_On_1+86400*4  OutDataTypeStr=boolean
  Interval Test1 : simulink/Logic and Bit Operations/Interval Test  IntervalClosedRight=on  uplimit=K_L1_Off_2+86400*4  IntervalClosedLeft=on  lowlimit=K_L1_On_2+86400*4  OutDataTypeStr=boolean
  Switch : Switch  Criteria=u2 > Threshold  Threshold=0.5
  Switch1 : Switch  Criteria=u2 > Threshold  Threshold=0.5
  Out1 : Outport  VectorParamsAs1DForOutWhenUnconnected=off
  wires:
  Clock/1 -> Gain/1
  Interval Test/1 -> Switch/2
  Switch/1 -> Add/1
  Interval Test1/1 -> Switch1/2
  Add/1 -> Out1/1
  Constant1/1 -> Switch/3, Switch1/3
  Constant/1 -> Switch/1, Switch1/1
  Switch1/1 -> Add/2
  Gain/1 -> Interval Test1/1, Interval Test/1

== system Microgrid_W/House 5 W1/Light 1/D6 ==
  Add : Sum
  Clock : Clock
  Constant : Constant
  Constant1 : Constant  Value=0
  Gain : Gain  Gain=t
  Interval Test : simulink/Logic and Bit Operations/Interval Test  IntervalClosedRight=on  uplimit=K_L1_Off_1+86400*5  IntervalClosedLeft=on  lowlimit=K_L1_On_1+86400*5  OutDataTypeStr=boolean
  Interval Test1 : simulink/Logic and Bit Operations/Interval Test  IntervalClosedRight=on  uplimit=K_L1_Off_2+86400*5  IntervalClosedLeft=on  lowlimit=K_L1_On_2+86400*5  OutDataTypeStr=boolean
  Switch : Switch  Criteria=u2 > Threshold  Threshold=0.5
  Switch1 : Switch  Criteria=u2 > Threshold  Threshold=0.5
  Out1 : Outport  VectorParamsAs1DForOutWhenUnconnected=off
  wires:
  Clock/1 -> Gain/1
  Gain/1 -> Interval Test/1, Interval Test1/1
  Switch1/1 -> Add/2
  Constant/1 -> Switch1/1, Switch/1
  Constant1/1 -> Switch1/3, Switch/3
  Add/1 -> Out1/1
  Interval Test1/1 -> Switch1/2
  Switch/1 -> Add/1
  Interval Test/1 -> Switch/2

== system Microgrid_W/House 5 W1/Light 1/D7 ==
  Add : Sum
  Clock : Clock
  Constant : Constant
  Constant1 : Constant  Value=0
  Gain : Gain  Gain=t
  Interval Test : simulink/Logic and Bit Operations/Interval Test  IntervalClosedRight=on  uplimit=K_L1_Off_1+86400*6  IntervalClosedLeft=on  lowlimit=K_L1_On_1+86400*6  OutDataTypeStr=boolean
  Interval Test1 : simulink/Logic and Bit Operations/Interval Test  IntervalClosedRight=on  uplimit=K_L1_Off_2+86400*6  IntervalClosedLeft=on  lowlimit=K_L1_On_2+86400*6  OutDataTypeStr=boolean
  Switch : Switch  Criteria=u2 > Threshold  Threshold=0.5
  Switch1 : Switch  Criteria=u2 > Threshold  Threshold=0.5
  Out1 : Outport  VectorParamsAs1DForOutWhenUnconnected=off
  wires:
  Clock/1 -> Gain/1
  Interval Test/1 -> Switch/2
  Switch/1 -> Add/1
  Interval Test1/1 -> Switch1/2
  Add/1 -> Out1/1
  Constant1/1 -> Switch/3, Switch1/3
  Constant/1 -> Switch/1, Switch1/1
  Switch1/1 -> Add/2
  Gain/1 -> Interval Test1/1, Interval Test/1

== system Microgrid_W/House 5 W1/Light 2/D1 ==
  Add : Sum
  Clock : Clock
  Compare To Zero : simulink/Logic and Bit Operations/Compare To Zero  relop=>  OutDataTypeStr=boolean
  Compare To Zero1 : simulink/Logic and Bit Operations/Compare To Zero  relop=>  OutDataTypeStr=boolean
  Constant : Constant
  Constant1 : Constant  Value=0
  Constant2 : Constant  Value=0
  Constant3 : Constant  Value=Dishwasher_On
  Constant4 : Constant
  Constant5 : Constant  Value=0
  Constant6 : Constant  Value=Dishwasher_On
  Gain : Gain  Gain=t
  Interval Test : simulink/Logic and Bit Operations/Interval Test  IntervalClosedRight=on  uplimit=Dishwasher_On+23  IntervalClosedLeft=on  lowlimit=Dishwasher_On+13  OutDataTypeStr=boolean
  Interval Test1 : simulink/Logic and Bit Operations/Interval Test  IntervalClosedRight=on  uplimit=Dishwasher_On+66  IntervalClosedLeft=on  lowlimit=Dishwasher_On+52  OutDataTypeStr=boolean
  Switch{,1..2,4} (4 alike) : Switch  Criteria=u2 > Threshold  Threshold=0.5
  Out1 : Outport  VectorParamsAs1DForOutWhenUnconnected=off
  wires:
  Clock/1 -> Gain/1
  Add/1 -> Out1/1
  Switch2/1 -> Add/2
  Switch/1 -> Add/1
  Switch4/1 -> Switch2/1
  Compare To Zero1/1 -> Switch4/2
  Constant5/1 -> Switch4/3
  Constant4/1 -> Switch4/1
  Constant6/1 -> Compare To Zero1/1
  Interval Test1/1 -> Switch2/2
  Switch1/1 -> Switch/1
  Compare To Zero/1 -> Switch1/2
  Constant2/1 -> Switch1/3
  Constant/1 -> Switch1/1
  Constant3/1 -> Compare To Zero/1
  Gain/1 -> Interval Test1/1, Interval Test/1
  Constant1/1 -> Switch/3, Switch2/3
  Interval Test/1 -> Switch/2
